simulink model "canyongenerator"  (Simulink 8.9)
settings: Solver=ode45  StartTime=0.0  StopTime=6000  RelTol=1e-3  EnableMultiTasking=on
settings Model: Creator=tlombaerts  LastModifiedBy=TUDelft SID
settings DataIOCC: LimitDataPoints=off
settings OptimizationCC: ExpressionDepthLimit=2147483647  InitFltsAndDblsToZero=on
settings DebuggingCC: SaveWithParameterizedLinksMsg=none  UnderspecifiedInitializationDetection=Simplified  MergeDetectMultiDrivingBlocksExec=error  SignalResolutionControl=TryResolveAllWithWarning  SolverPrmCheckMsg=warning
settings GRTTargetCC: TargetFcnLib=ansi_tfl_tmw.mat  GeneratePreprocessorConditionals=Use local settings

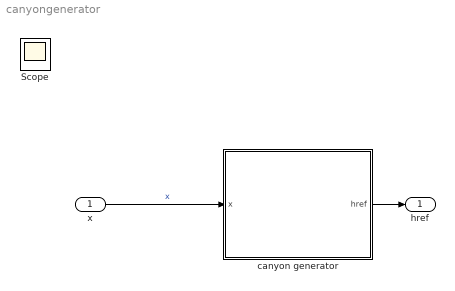
== system canyongenerator ==
  x : Inport
  canyon generator : Subsystem
      mask Display: image(imread('refalt.jpg'))
  href : Outport
  Scope : Scope
  wires:
  x/1 -> canyon generator/1(x)  "x"
  canyon generator/1(href) -> href/1

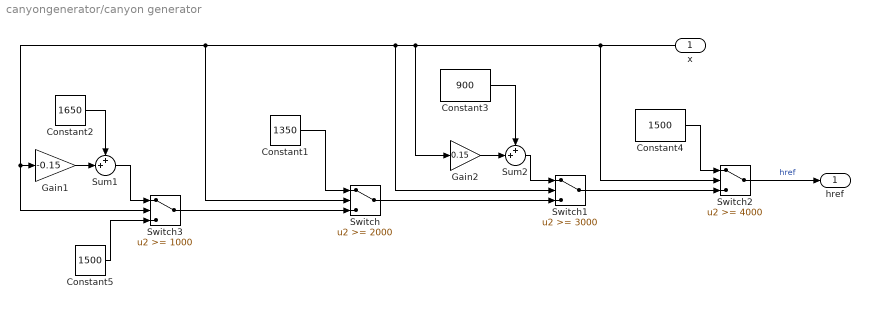
== system canyongenerator/canyon generator ==
  x : Inport
  Constant1 : Constant  Value=1350
  Constant2 : Constant  Value=1650
  Constant3 : Constant  Value=900
  Constant4 : Constant  Value=1500
  Constant5 : Constant  Value=1500
  Gain1 : Gain  Gain=-0.15
  Gain2 : Gain  Gain=0.15
  Sum1 : Sum  Inputs=++|
  Sum2 : Sum  Inputs=++|
  Switch : Switch  Threshold=2000  ZeroCross=off
  Switch1 : Switch  Threshold=3000  ZeroCross=off
  Switch2 : Switch  Threshold=4000  ZeroCross=off
  Switch3 : Switch  Threshold=1000  ZeroCross=off
  href : Outport
  wires:
  Constant1/1 -> Switch/1
  x/1 -> Switch2/2, Gain2/1, Switch1/2, Switch/2, Gain1/1, Switch3/2
  Switch/1 -> Switch1/3
  Gain2/1 -> Sum2/2
  Constant3/1 -> Sum2/1
  Sum2/1 -> Switch1/1
  Switch1/1 -> Switch2/3
  Constant4/1 -> Switch2/1
  Switch2/1 -> href/1  "href"
  Switch3/1 -> Switch/3
  Constant5/1 -> Switch3/3
  Sum1/1 -> Switch3/1
  Gain1/1 -> Sum1/2
  Constant2/1 -> Sum1/1
